simulink model "lab7"  (R2016a)
settings: Solver=VariableStepAuto  StartTime=0.0  StopTime=10.0  RelTol=1e-3
undefined symbols (not defined in the file): DiscIntNeverNeededParam
libraries: dsparch4 x1, commsynccomp2 x1, dspsrcs4 x1
settings Model: Creator=User  LastModifiedBy=User

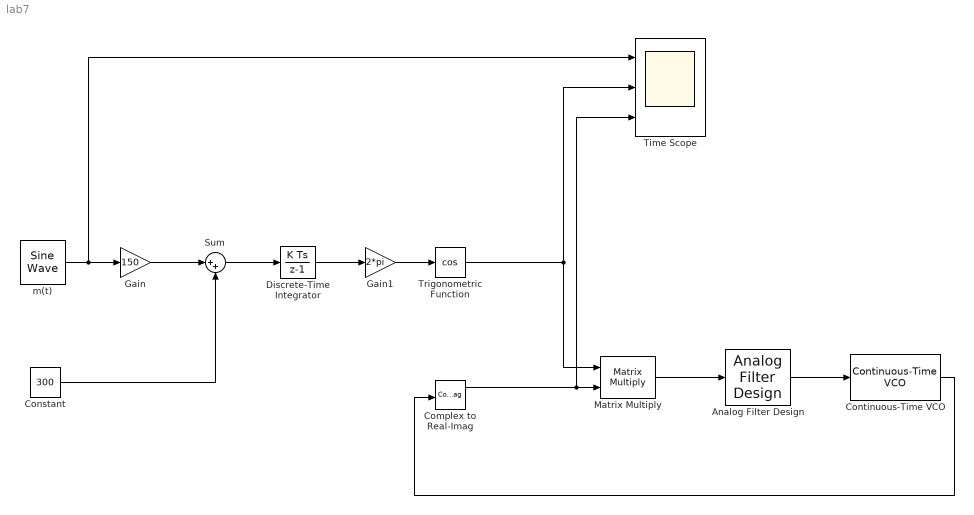
== system lab7 ==
  Analog Filter Design : dsparch4/Analog Filter Design  method=Butterworth  filttype=Lowpass  N=10  Wlo=2*pi*10  Whi=80  Rp=2  Rs=40
  Complex to Real-Imag : ComplexToRealImag
  Constant : Constant  Value=300
  Continuous-Time VCO : commsynccomp2/Continuous-Time VCO  Ac=1  Fc=10  Kc=50  Ph=0
  Discrete-Time Integrator : DiscreteIntegrator  InitialConditionSetting=State (most efficient)  SampleTime=1/98000  ICPrevOutput=DiscIntNeverNeededParam  ICPrevScaledInput=DiscIntNeverNeededParam
  Gain : Gain  Gain=150
  Gain1 : Gain  Gain=2*pi
  Matrix Multiply : Product  Multiplication=Matrix(*)
  Sum : Sum  Inputs=|++  RndMeth=Round
  Time Scope : Scope  NumInputPorts=3
  Trigonometric Function : Trigonometry  Operator=cos
  m(t) : dspsrcs4/Sine Wave  Amplitude=1  Frequency=10  Phase=90  SampleMode=Discrete  OutComplex=Real  CompMethod=Trigonometric fcn  TableSize=Speed  SampleTime=1/98000  SamplesPerFrame=1  ResetState=Restart at time zero  OutputFrames=off  dataType=double  wordLen=16  udDataType=sfix(16)  fracBitsMode=Best precision  numFracBits=15  OutDataTypeStr=double  LastOutDataTypeStr=double
  wires:
  Gain/1 -> Sum/1
  Constant/1 -> Sum/2
  Gain1/1 -> Trigonometric Function/1
  Sum/1 -> Discrete-Time Integrator/1
  Discrete-Time Integrator/1 -> Gain1/1
  m(t)/1 -> Time Scope/1, Gain/1
  Trigonometric Function/1 -> Time Scope/2, Matrix Multiply/1
  Continuous-Time VCO/1 -> Complex to Real-Imag/1
  Complex to Real-Imag/1 -> Time Scope/3, Matrix Multiply/2
  Matrix Multiply/1 -> Analog Filter Design/1
  Analog Filter Design/1 -> Continuous-Time VCO/1
